simulink model "Question10_AkankshaMurali"  (R2023b)
settings: Solver=VariableStepAuto  StartTime=0.0  StopTime=10.0  RelTol=1e-3
settings Model: Creator=akank  LastModifiedBy=akank

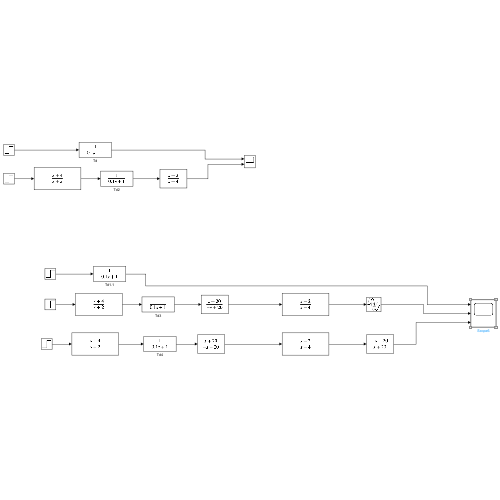
[thumbnail: Simulink's stored preview of the top-level diagram]
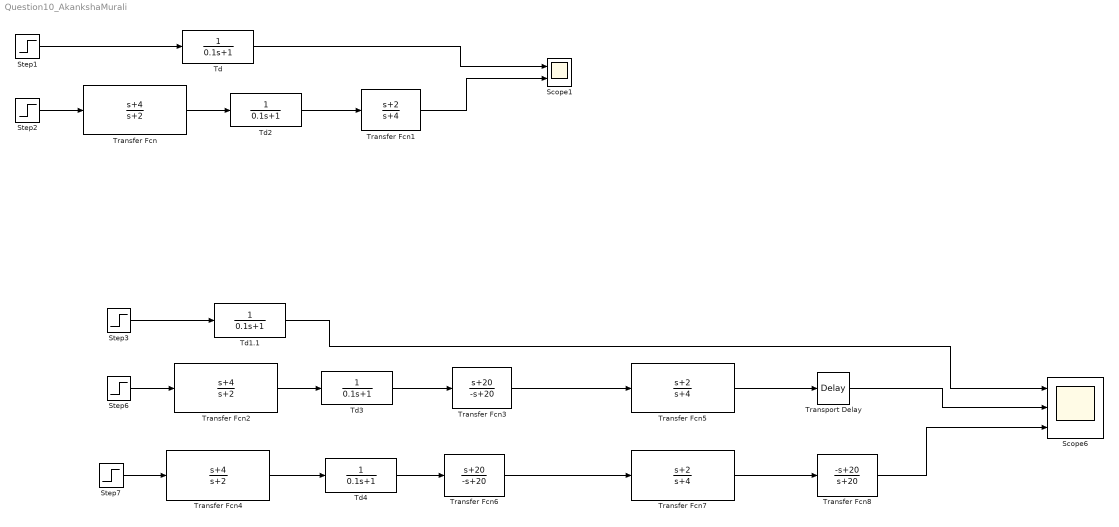
== system Question10_AkankshaMurali ==
  Scope1 : Scope  NumInputPorts=2
  Scope6 : Scope  NumInputPorts=3
  Step{1..3,6..7} (5 alike) : Step  Time=0  SampleTime=0
  Td{,2..4} (4 alike) : TransferFcn  Denominator=[0.1 1]
  Td1.1 : TransferFcn  Denominator=[0.1 1]
  Transfer Fcn : TransferFcn  Numerator=[1 4]  Denominator=[1 2]
  Transfer Fcn1 : TransferFcn  Numerator=[1 2]  Denominator=[1 4]
  Transfer Fcn2 : TransferFcn  Numerator=[1 4]  Denominator=[1 2]
  Transfer Fcn3 : TransferFcn  Numerator=[1 20]  Denominator=[-1 20]
  Transfer Fcn4 : TransferFcn  Numerator=[1 4]  Denominator=[1 2]
  Transfer Fcn5 : TransferFcn  Numerator=[1 2]  Denominator=[1 4]
  Transfer Fcn6 : TransferFcn  Numerator=[1 20]  Denominator=[-1 20]
  Transfer Fcn7 : TransferFcn  Numerator=[1 2]  Denominator=[1 4]
  Transfer Fcn8 : TransferFcn  Numerator=[-1 20]  Denominator=[1 20]
  Transport Delay : TransportDelay  DelayTime=0.1
  wires:
  Td4/1 -> Transfer Fcn6/1
  Transfer Fcn6/1 -> Transfer Fcn7/1
  Td/1 -> Scope1/1
  Transfer Fcn8/1 -> Scope6/3
  Transport Delay/1 -> Scope6/2
  Td2/1 -> Transfer Fcn1/1
  Transfer Fcn5/1 -> Transport Delay/1
  Transfer Fcn4/1 -> Td4/1
  Transfer Fcn2/1 -> Td3/1
  Step7/1 -> Transfer Fcn4/1
  Transfer Fcn3/1 -> Transfer Fcn5/1
  Step3/1 -> Td1.1/1
  Td1.1/1 -> Scope6/1
  Td3/1 -> Transfer Fcn3/1
  Transfer Fcn7/1 -> Transfer Fcn8/1
  Transfer Fcn1/1 -> Scope1/2
  Transfer Fcn/1 -> Td2/1
  Step6/1 -> Transfer Fcn2/1
  Step1/1 -> Td/1
  Step2/1 -> Transfer Fcn/1
